simulink model "Cruise_Control"  (R2020b)
settings: Solver=ode45  StartTime=0.0  StopTime=120  RelTol=1e-3
values from neighbouring files (symbols this model uses):
  b = 50    [data.mat]
  m = 1000    [data.mat]
settings Model: DataDictionary=Data1.sldd  Creator=vijay jagtap  LastModifiedBy=vijay jagtap
settings SolverCC: MaxConsecutiveMinStep=1000

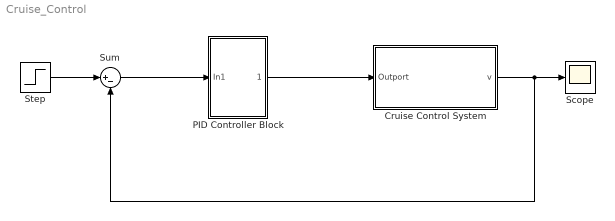
== system Cruise_Control ==
  Cruise Control System : Subsystem
  PID Controller Block : Subsystem
  Scope : Scope
  Step : Step  Time=0  After=u  SampleTime=0
  Sum : Sum  Inputs=|+-
  wires:
  Step/1 -> Sum/1
  Cruise Control System/1(v) -> Sum/2, Scope/1
  PID Controller Block/1(Outport) -> Cruise Control System/1(Outport)
  Sum/1 -> PID Controller Block/1(In1)

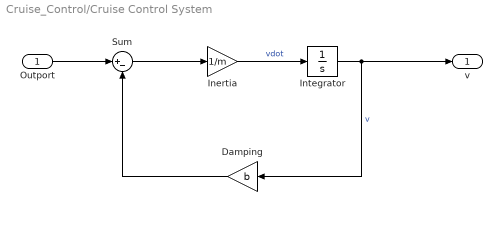
== system Cruise_Control/Cruise Control System ==
  Outport : Inport
  Damping : Gain  Gain=b
  Inertia : Gain  Gain=1/m
  Integrator : Integrator
  Sum : Sum  Inputs=|+-
  v : Outport
  wires:
  Inertia/1 -> Integrator/1  "vdot"
  Integrator/1 -> v/1, Damping/1  "v"
  Damping/1 -> Sum/2
  Sum/1 -> Inertia/1
  Outport/1 -> Sum/1

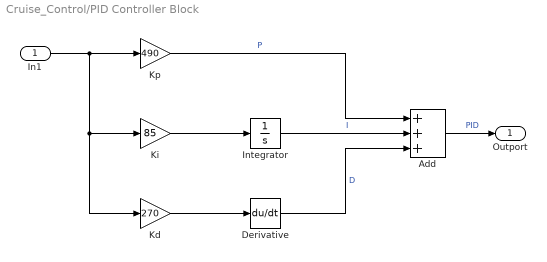
== system Cruise_Control/PID Controller Block ==
  In1 : Inport
  Add : Sum  Inputs=+++
  Derivative : Derivative
  Integrator : Integrator
  Kd : Gain  Gain=270
  Ki : Gain  Gain=85
  Kp : Gain  Gain=490
  Outport : Outport
  wires:
  In1/1 -> Kd/1, Ki/1, Kp/1
  Kd/1 -> Derivative/1
  Kp/1 -> Add/1  "P"
  Ki/1 -> Integrator/1
  Derivative/1 -> Add/3  "D"
  Integrator/1 -> Add/2  "I"
  Add/1 -> Outport/1  "PID"
